simulink model "ex_4"  (R2020b)
settings: Solver=ode23tb  StartTime=0.0  StopTime=20e3  MaxStep=1  RelTol=1e-3
libraries: component_lib x22, pid_lib x2
settings Model: Creator=maxjo65  LastModifiedBy=maxjo65

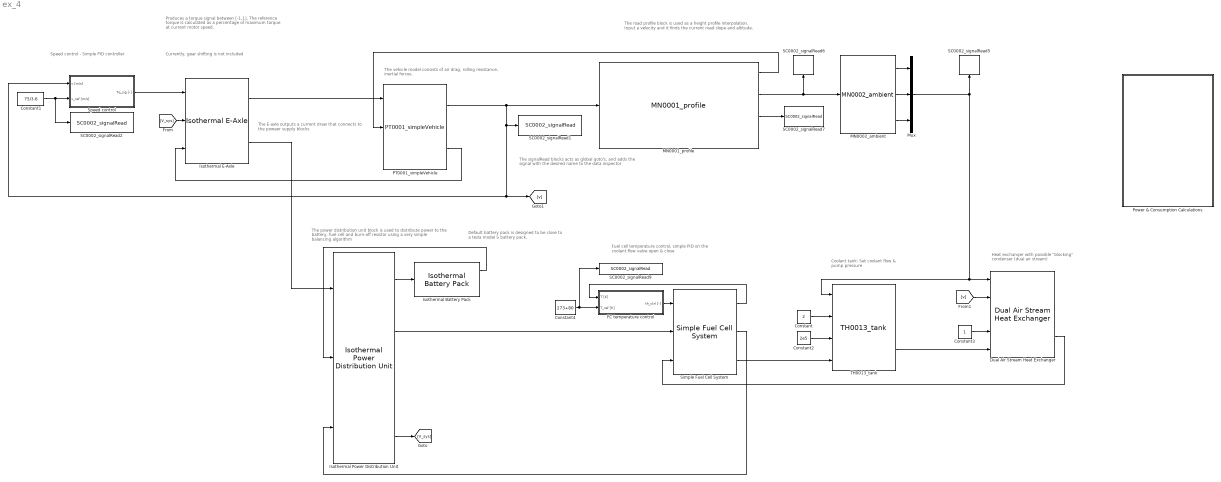
== system ex_4 ==
  note: The power distribution unit block is used
      | to distribute power to the battery, fuel cell and burn-off resistor
      | using a very simple balancing algorithm
  note: The road profile block is used as a height profile interpolation.
      | Input a velocity and it finds the current road slope and altitude.
  note: The vehicle model consists of air drag, rolling resistance,
      | inertial forces.
  note: Currently, gear shifting is not included
  note: Produces a torque signal between [-1,1].
      |
      | The reference torque is calculated as a percentage of
      | maximum torque at current motor speed.
  note: Speed control - Simple PID controller
  note: The signalRead blocks acts as global goto's, and adds the signal with the desired name to the data inspector
  note: The E-axle outputs a current draw that connects
      | to the poweer supply blocks
  note: Default battery pack is designed to be close
      | to a tesla model S battery pack.
  note: Fuel cell temperature control,
      | simple PID on the coolant flow valve open & close
  note: Coolant tank:
      | Set coolant flow & pump pressure
  note: Heat exchanger with possible
      | "blocking" condenser (dual air stream)
  Constant : Constant  Value=2
  Constant1 : Constant  Value=75/3.6
  Constant2 : Constant  Value=2e5
  Constant3 : Constant
  Constant4 : Constant  Value=273+80
  Dual Air Stream Heat Exchanger : component_lib/Dual Air Stream Heat Exchanger  HtH=1.1  StS=0.95
  FC temperature control : Subsystem
  Isothermal Battery Pack : component_lib/Isothermal Battery Pack  SOC_0=0.5  n_mod_ser=16  n_mod_par=1
  Isothermal E-Axle : component_lib/Isothermal E-Axle  n=2
  Isothermal Power Distribution Unit : component_lib/Isothermal Power Distribution Unit  V_sys=420  P_fc=80e3  I_bt_max=300  I_bt_min=-200  T_s=1
  MN0001_profile : component_lib/Mission/MN0001_profile  profile=Sodertalje_Norrkoping.mat  x0=0  N_lookahead=100
  MN0002_ambient : component_lib/Mission/MN0002_ambient  p_0=1.01e5  T_0=273 + 20  RH_0=0.2
  Mux : Mux  Inputs=3
  PT0001_simpleVehicle : component_lib/Powertrain/PT0001_simpleVehicle  m=20e3  r_w=0.5  A_f=10  C_d=0.5  rho_air=1.225  c_r0=0.0060  c_r1=2.3e-7  gain=600  v0=75/3.6  x0=0
  Power & Consumption Calculations : Subsystem
  SC0002_signalRead1 : component_lib/Data & Control/SC0002_signalRead  SigName=velocity
  SC0002_signalRead2 : component_lib/Data & Control/SC0002_signalRead  SigName=velocityReference
  SC0002_signalRead5 : component_lib/Data & Control/SC0002_signalRead  SigName=ambient
  SC0002_signalRead6 : component_lib/Data & Control/SC0002_signalRead  SigName=altitude
  SC0002_signalRead7 : component_lib/Data & Control/SC0002_signalRead  SigName=distance
  SC0002_signalRead9 : component_lib/Data & Control/SC0002_signalRead  SigName=fuelCellTemperatureReference
  Simple Fuel Cell System : component_lib/Simple Fuel Cell System  n_st=2
  Speed control : Subsystem
  TH0013_tank : component_lib/Thermal Systems/TH0013_tank  V=5e-3
  wires:
  [V_sys] -> Isothermal E-Axle/2
  Isothermal E-Axle/1 -> PT0001_simpleVehicle/1
  PT0001_simpleVehicle/2 -> Isothermal E-Axle/3
  Speed control/1(Tq_sig [-]) -> Isothermal E-Axle/1
  Constant1/1 -> Speed control/2(v_ref [m/s]), SC0002_signalRead2/1
  MN0001_profile/1 -> PT0001_simpleVehicle/2
  PT0001_simpleVehicle/1 -> Speed control/1(v [m/s]), [v], SC0002_signalRead1/1, MN0001_profile/1
  Isothermal E-Axle/2 -> Isothermal Power Distribution Unit/1
  Isothermal Power Distribution Unit/1 -> Isothermal Battery Pack/1
  Isothermal Battery Pack/1 -> Isothermal Power Distribution Unit/2
  Isothermal Power Distribution Unit/2 -> Simple Fuel Cell System/2
  Simple Fuel Cell System/2 -> Isothermal Power Distribution Unit/3
  Isothermal Power Distribution Unit/4 -> [V_sys]
  Simple Fuel Cell System/3 -> TH0013_tank/4
  TH0013_tank/2 -> Dual Air Stream Heat Exchanger/5
  Dual Air Stream Heat Exchanger/2 -> Simple Fuel Cell System/3
  Constant/1 -> TH0013_tank/2
  Constant2/1 -> TH0013_tank/3
  MN0002_ambient/3 -> Mux/3
  MN0002_ambient/1 -> Mux/1
  MN0001_profile/2 -> MN0002_ambient/1, SC0002_signalRead6/1
  Mux/1 -> SC0002_signalRead5/1, TH0013_tank/1, Dual Air Stream Heat Exchanger/1
  MN0002_ambient/2 -> Mux/2
  MN0001_profile/3 -> SC0002_signalRead7/1
  FC temperature control/1(th_ctrl [-]) -> Simple Fuel Cell System/1
  Constant4/1 -> SC0002_signalRead9/1, FC temperature control/2(T_ref [K])
  Simple Fuel Cell System/1 -> FC temperature control/1(T [K])
  Constant3/1 -> Dual Air Stream Heat Exchanger/4
  [v] -> Dual Air Stream Heat Exchanger/2

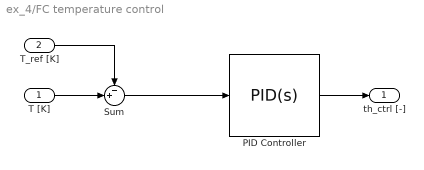
== system ex_4/FC temperature control ==
  T [K] : Inport
  T_ref [K] : Inport  Port=2
  PID Controller : pid_lib/PID Controller  Controller=PID  Form=Parallel  TimeDomain=Continuous-time  UseExternalTs=off  SampleTime=-1  IntegratorMethod=Forward Euler  FilterMethod=Forward Euler  ControllerParametersSource=internal  P=1e-2  I=1e-3  D=0  UseFilter=on  N=100  TunerSelectOption=Transfer Function Based (PID Tuner App)  InitialConditionSource=internal  InitialConditionForIntegrator=0  InitialConditionForFilter=0  DifferentiatorICPrevScaledInput=0  ExternalReset=none  TrackingMode=off  Kt=1  LimitOutput=on  SatLimitsSource=internal  UpperSaturationLimit=1  LowerSaturationLimit=0  LinearizeAsGain=on  AntiWindupMode=clamping  Kb=1  POutMin=[]  POutMax=[]  IOutMin=[]  IOutMax=[]  DOutMin=[]  DOutMax=[]  NOutMin=[]  NOutMax=[]  SumOutMin=[]  SumOutMax=[]  SaturationOutMin=[]  SaturationOutMax=[]  PParamMin=[]  PParamMax=[]  IParamMin=[]  IParamMax=[]  DParamMin=[]  DParamMax=[]  NParamMin=[]  NParamMax=[]  KbParamMin=[]  KbParamMax=[]  KtParamMin=[]  KtParamMax=[]  KbOutMin=[]  KbOutMax=[]  KtOutMin=[]  KtOutMax=[]  IntegratorOutMin=[]  IntegratorOutMax=[]  FilterOutMin=[]  FilterOutMax=[]  SumI1OutMin=[]  SumI1OutMax=[]  SumI2OutMin=[]  SumI2OutMax=[]  SumI3OutMin=[]  SumI3OutMax=[]  SumI4OutMin=[]  SumI4OutMax=[]  SumDOutMin=[]  SumDOutMax=[]  DifferentiatorOutMin=[]  DifferentiatorOutMax=[]  FilterDiffOutCoefMin=[]  FilterDiffOutCoefMax=[]  ReciprocalOutMin=[]  ReciprocalOutMax=[]  SumDenOutMin=[]  SumDenOutMax=[]  SumNumOutMin=[]  SumNumOutMax=[]  DivideOutMin=[]  DivideOutMax=[]  UdiffTsProdOutMin=[]  UdiffTsProdOutMax=[]  NTsProdOutMin=[]  NTsProdOutMax=[]  UintegralTsProdOutMin=[]  UintegralTsProdOutMax=[]  UngainTsProdOutMin=[]  UngainTsProdOutMax=[]  IntegratorContinuousStateAttributes=''  IntegratorStateMustResolveToSignalObject=off  IntegratorRTWStateStorageClass=Auto  FilterContinuousStateAttributes=''  FilterStateMustResolveToSignalObject=off  FilterRTWStateStorageClass=Auto  ParallelPVariant=InternalParameters  IdealPVariant=Disabled  IVariant=InternalParameters  DVariant=InternalParameters  IntegratorVariant=Continuous  SatVariant=Enabled  AWVariant=ContClampingParallel  PCopyVariant=Disabled  TRVariant=Disabled  FdbkBlocksVariant=Forward  IdealPFdbkVariant=Disabled  SatFdbkVariant=Disabled  DerivativeFilterVariant=ContFilter  NVariant=InternalParameters  NCopyVariant=Disabled  FilterICVariant=InternalICsFilter  IntegratorICVariant=InternalICs  ExternalResetVariant=Disabled  TRSumVariant=Passthrough  SumFdbkVariant=Disabled  SumVariant=Sum_PID  TsampFilterVariant=InternalTs  TsampNgainVariant=Passthrough  TsampIntegralVariant=Passthrough  ExternalSaturationOutDataTypeStr=Inherit: Same as second input
  Sum : Sum  Inputs=-+|
  th_ctrl [-] : Outport
  wires:
  PID Controller/1 -> th_ctrl [-]/1
  T_ref [K]/1 -> Sum/1
  T [K]/1 -> Sum/2
  Sum/1 -> PID Controller/1

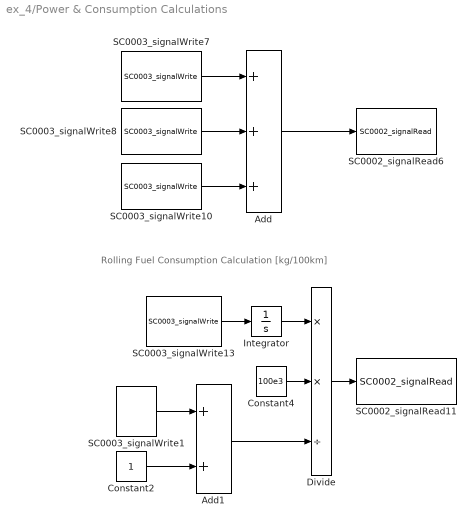
== system ex_4/Power & Consumption Calculations ==
  note: Rolling Fuel Consumption Calculation [kg/100km]
  Add : Sum  Inputs=+++
  Add1 : Sum
  Constant2 : Constant
  Constant4 : Constant  Value=100e3
  Divide : Product  Inputs=**/
  Integrator : Integrator
  SC0002_signalRead11 : component_lib/Data & Control/SC0002_signalRead  SigName=fuelConsumption
  SC0002_signalRead6 : component_lib/Data & Control/SC0002_signalRead  SigName=producedPower
  SC0003_signalWrite1 : component_lib/Data & Control/SC0003_signalWrite  SigName=distance
  SC0003_signalWrite10 : component_lib/Data & Control/SC0003_signalWrite  SigName=burnOffPower
  SC0003_signalWrite13 : component_lib/Data & Control/SC0003_signalWrite  SigName=hydrogenFlow
  SC0003_signalWrite7 : component_lib/Data & Control/SC0003_signalWrite  SigName=batteryPower
  SC0003_signalWrite8 : component_lib/Data & Control/SC0003_signalWrite  SigName=fuelCellPower
  wires:
  Integrator/1 -> Divide/1
  SC0003_signalWrite7/1 -> Add/1
  SC0003_signalWrite10/1 -> Add/3
  SC0003_signalWrite1/1 -> Add1/1
  SC0003_signalWrite8/1 -> Add/2
  Add/1 -> SC0002_signalRead6/1
  Add1/1 -> Divide/3
  Constant4/1 -> Divide/2
  Constant2/1 -> Add1/2
  Divide/1 -> SC0002_signalRead11/1
  SC0003_signalWrite13/1 -> Integrator/1

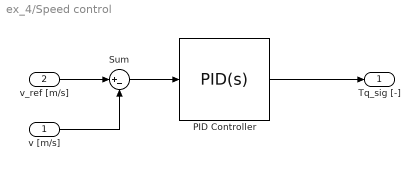
== system ex_4/Speed control ==
  v [m/s] : Inport
  v_ref [m/s] : Inport  Port=2
  PID Controller : pid_lib/PID Controller  Controller=PID  Form=Parallel  TimeDomain=Continuous-time  UseExternalTs=off  SampleTime=-1  IntegratorMethod=Forward Euler  FilterMethod=Forward Euler  ControllerParametersSource=internal  P=10  I=1e-1  D=0  UseFilter=on  N=100  TunerSelectOption=Transfer Function Based (PID Tuner App)  InitialConditionSource=internal  InitialConditionForIntegrator=0  InitialConditionForFilter=0  DifferentiatorICPrevScaledInput=0  ExternalReset=none  TrackingMode=off  Kt=1  LimitOutput=on  SatLimitsSource=internal  UpperSaturationLimit=1  LowerSaturationLimit=-1  LinearizeAsGain=on  AntiWindupMode=clamping  Kb=1  POutMin=[]  POutMax=[]  IOutMin=[]  IOutMax=[]  DOutMin=[]  DOutMax=[]  NOutMin=[]  NOutMax=[]  SumOutMin=[]  SumOutMax=[]  SaturationOutMin=[]  SaturationOutMax=[]  PParamMin=[]  PParamMax=[]  IParamMin=[]  IParamMax=[]  DParamMin=[]  DParamMax=[]  NParamMin=[]  NParamMax=[]  KbParamMin=[]  KbParamMax=[]  KtParamMin=[]  KtParamMax=[]  KbOutMin=[]  KbOutMax=[]  KtOutMin=[]  KtOutMax=[]  IntegratorOutMin=[]  IntegratorOutMax=[]  FilterOutMin=[]  FilterOutMax=[]  SumI1OutMin=[]  SumI1OutMax=[]  SumI2OutMin=[]  SumI2OutMax=[]  SumI3OutMin=[]  SumI3OutMax=[]  SumI4OutMin=[]  SumI4OutMax=[]  SumDOutMin=[]  SumDOutMax=[]  DifferentiatorOutMin=[]  DifferentiatorOutMax=[]  FilterDiffOutCoefMin=[]  FilterDiffOutCoefMax=[]  ReciprocalOutMin=[]  ReciprocalOutMax=[]  SumDenOutMin=[]  SumDenOutMax=[]  SumNumOutMin=[]  SumNumOutMax=[]  DivideOutMin=[]  DivideOutMax=[]  UdiffTsProdOutMin=[]  UdiffTsProdOutMax=[]  NTsProdOutMin=[]  NTsProdOutMax=[]  UintegralTsProdOutMin=[]  UintegralTsProdOutMax=[]  UngainTsProdOutMin=[]  UngainTsProdOutMax=[]  IntegratorContinuousStateAttributes=''  IntegratorStateMustResolveToSignalObject=off  IntegratorRTWStateStorageClass=Auto  FilterContinuousStateAttributes=''  FilterStateMustResolveToSignalObject=off  FilterRTWStateStorageClass=Auto  ParallelPVariant=InternalParameters  IdealPVariant=Disabled  IVariant=InternalParameters  DVariant=InternalParameters  IntegratorVariant=Continuous  SatVariant=Enabled  AWVariant=ContClampingParallel  PCopyVariant=Disabled  TRVariant=Disabled  FdbkBlocksVariant=Forward  IdealPFdbkVariant=Disabled  SatFdbkVariant=Disabled  DerivativeFilterVariant=ContFilter  NVariant=InternalParameters  NCopyVariant=Disabled  FilterICVariant=InternalICsFilter  IntegratorICVariant=InternalICs  ExternalResetVariant=Disabled  TRSumVariant=Passthrough  SumFdbkVariant=Disabled  SumVariant=Sum_PID  TsampFilterVariant=InternalTs  TsampNgainVariant=Passthrough  TsampIntegralVariant=Passthrough  ExternalSaturationOutDataTypeStr=Inherit: Same as second input
  Sum : Sum  Inputs=|+-
  Tq_sig [-] : Outport
  wires:
  PID Controller/1 -> Tq_sig [-]/1
  Sum/1 -> PID Controller/1
  v_ref [m/s]/1 -> Sum/1
  v [m/s]/1 -> Sum/2
